simulink model "MotorCtrl_FOC_Physic"  (R2023b)
settings: Solver=FixedStepDiscrete  StartTime=0.0  StopTime=10  FixedStep=MC_Sim_BaseStep  RelTol=1e-3  EnableMultiTasking=on
values from neighbouring files (symbols this model uses):
  MC_MOS_DeadTime = 1.0E-6    [MotorControlDataDictionary_Math.sldd]    (also in MotorControlDataDictionary_Physic.sldd)
  MC_Motor_Mechinal_Inertia = 0.0103    [MotorControlDataDictionary_Math.sldd]    (also in MotorControlDataDictionary_Physic.sldd)
  MC_Motor_Phi = 0.0059190254913385806    [MotorControlDataDictionary_Math.sldd]    (also in MotorControlDataDictionary_Physic.sldd)
  MC_Motor_Rotor_Pn = 4.0    [MotorControlDataDictionary_Math.sldd]    (also in MotorControlDataDictionary_Physic.sldd)
  MC_Motor_Stator_Ld = 5.6345E-5    [MotorControlDataDictionary_Math.sldd]    (also in MotorControlDataDictionary_Physic.sldd)
  MC_Motor_Stator_Lq = 5.6345E-5    [MotorControlDataDictionary_Math.sldd]    (also in MotorControlDataDictionary_Physic.sldd)
  MC_Motor_Stator_Rs = 0.0286    [MotorControlDataDictionary_Math.sldd]    (also in MotorControlDataDictionary_Physic.sldd)
  MC_Param_CurrentPI_Ki = 0.0071879639914134473    [MotorControlDataDictionary_Math.sldd]    (also in MotorControlDataDictionary_Physic.sldd)
  MC_Param_CurrentPI_Kp = 0.283220860906427    [MotorControlDataDictionary_Math.sldd]    (also in MotorControlDataDictionary_Physic.sldd)
  MC_Param_CurrentPI_UdInteMax = 7.794228634059948    [MotorControlDataDictionary_Math.sldd]    (also in MotorControlDataDictionary_Physic.sldd)
  MC_Param_CurrentPI_UdInteMin = -7.794228634059948    [MotorControlDataDictionary_Math.sldd]    (also in MotorControlDataDictionary_Physic.sldd)
  MC_Param_CurrentPI_UdMax = 7.794228634059948    [MotorControlDataDictionary_Math.sldd]    (also in MotorControlDataDictionary_Physic.sldd)
  MC_Param_CurrentPI_UdMin = -7.794228634059948    [MotorControlDataDictionary_Math.sldd]    (also in MotorControlDataDictionary_Physic.sldd)
  MC_Param_CurrentPI_UqInteMax = 7.794228634059948    [MotorControlDataDictionary_Math.sldd]    (also in MotorControlDataDictionary_Physic.sldd)
  MC_Param_CurrentPI_UqInteMin = -7.794228634059948    [MotorControlDataDictionary_Math.sldd]    (also in MotorControlDataDictionary_Physic.sldd)
  MC_Param_CurrentPI_UqMax = 7.794228634059948    [MotorControlDataDictionary_Math.sldd]    (also in MotorControlDataDictionary_Physic.sldd)
  MC_Param_CurrentPI_UqMin = -7.794228634059948    [MotorControlDataDictionary_Math.sldd]    (also in MotorControlDataDictionary_Physic.sldd)
  MC_Param_Flux_Gamma = 750000.0    [MotorControlDataDictionary_Math.sldd]    (also in MotorControlDataDictionary_Physic.sldd)
  MC_Param_PhasetoReal = 500.0    [MotorControlDataDictionary_Math.sldd]    (also in MotorControlDataDictionary_Physic.sldd)
  MC_Param_SMO_CoffA = 0.97462064069571386    [MotorControlDataDictionary_Math.sldd]    (also in MotorControlDataDictionary_Physic.sldd)
  MC_Param_SMO_CoffB = 0.88739018546454884    [MotorControlDataDictionary_Math.sldd]    (also in MotorControlDataDictionary_Physic.sldd)
  MC_Param_SpeedCtrl_IdMax = 60.0    [MotorControlDataDictionary_Math.sldd]    (also in MotorControlDataDictionary_Physic.sldd)
  MC_Param_SpeedCtrl_IdMin = -60.0    [MotorControlDataDictionary_Math.sldd]    (also in MotorControlDataDictionary_Physic.sldd)
  MC_Param_SpeedCtrl_IqMax = 60.0    [MotorControlDataDictionary_Math.sldd]    (also in MotorControlDataDictionary_Physic.sldd)
  MC_Param_SpeedCtrl_IqMin = -60.0    [MotorControlDataDictionary_Math.sldd]    (also in MotorControlDataDictionary_Physic.sldd)
  MC_Param_SpeedPI_Ki = 0.57248683633241571    [MotorControlDataDictionary_Math.sldd]    (also in MotorControlDataDictionary_Physic.sldd)
  MC_Param_SpeedPI_Kp = 9.1114109857344836    [MotorControlDataDictionary_Math.sldd]    (also in MotorControlDataDictionary_Physic.sldd)
  MC_Param_SpeedtoTheta = 5.0E-5    [MotorControlDataDictionary_Math.sldd]    (also in MotorControlDataDictionary_Physic.sldd)
  MC_Param_SVPWM_DutyMax = 0.98    [MotorControlDataDictionary_Math.sldd]    (also in MotorControlDataDictionary_Physic.sldd)
  MC_Param_SVPWM_DutyMin = 0.02    [MotorControlDataDictionary_Math.sldd]    (also in MotorControlDataDictionary_Physic.sldd)
  MC_Param_SVPWM_SampleOffset1 = 0.02    [MotorControlDataDictionary_Math.sldd]    (also in MotorControlDataDictionary_Physic.sldd)
  MC_Param_SVPWM_SampleOffset2 = 0.015    [MotorControlDataDictionary_Math.sldd]    (also in MotorControlDataDictionary_Physic.sldd)
  MC_Param_SVPWM_SampleValid = 0.011999999999999999    [MotorControlDataDictionary_Math.sldd]    (also in MotorControlDataDictionary_Physic.sldd)
  MC_Sample_CurrentNoise = 1.0E-15    [MotorControlDataDictionary_Math.sldd]    (also in MotorControlDataDictionary_Physic.sldd)
  MC_Sample_VbusNoise = 1.0E-15    [MotorControlDataDictionary_Math.sldd]    (also in MotorControlDataDictionary_Physic.sldd)
  MC_Sim_BaseStep = 5.0E-8    [MotorControlDataDictionary_Math.sldd]    (also in MotorControlDataDictionary_Physic.sldd)
  MC_Sim_HFTStep = 5.0E-5    [MotorControlDataDictionary_Math.sldd]    (also in MotorControlDataDictionary_Physic.sldd)
  MC_Sim_MFTStep = 0.002    [MotorControlDataDictionary_Math.sldd]    (also in MotorControlDataDictionary_Physic.sldd)
libraries: simulink x17, nesl_utility x15, ee_lib x10, fl_lib x8
(part 2 of 3)

== system MotorCtrl_FOC_Physic/Hardware_Math/MotorHardware ==
  Load : Inport
  PWM : Inport  Port=2
  Current and Voltage Sensor (Three-Phase) : ee_lib/Sensors & Transducers/Current and Voltage Sensor (Three-Phase)  vMeasurementType=ee.enum.vmeasurement.ll  outputUnit=ee.enum.unit.si  SRated=100e6 A*V  VRated=24e3 V  I_specify=off  I_priority=None  I=[0, 0, 0] A  I_nominal_specify=off  I_nominal_unit=A  I_nominal_value=1  V_specify=off  V_priority=None  V=[0, 0, 0] V  V_nominal_specify=off  V_nominal_unit=V  V_nominal_value=1
      settings: InternalSimscapePortConfiguration="{\"Bottom\":[],\"Left\":[{\"id\":\"a1\",\"label\":\"a1\",\"type\":\"foundation.electrical.electrical\"},{\"id\":\"b1\",\"label\":\"b1\",\"type\":\"foundation.electrical.electrical\"},{\"id\":\"c1\",\"label\":\"c1\",\"type\":\"foundation.electrical.electrical\"}],\"Right\":[{\"id\":\"V_output\",\"label\":\"V\",\"type\":\"output\"},{\"id\":\"I_output\",\"label\":\"I\",\"type\":\"output\"},{\"id\":\"a2\",\"label\":\"a2\",\"type\":\"foundation.electrical.electrical\"},{\"id\":\"b2\",\"label\":\"b2\",\"type\":\"foundation.electrical.electrical\"},{\"id\":\"c2\",\"label\":\"c2\",\"type\":\"foundation.electrical.electrical\"}],\"Top\":[]}"
  Demux : Demux  Outputs=6
  Electrical Reference : fl_lib/Electrical/Electrical Elements/Electrical Reference
  MOSFET (Ideal, Switching){,1..5} (6 alike) : ee_lib/Semiconductors & Converters/MOSFET (Ideal, Switching)  port_option=ee.enum.controlport.ps  Rds=MC_MOS_Rds Ohm  Goff=MC_MOS_Cs 1/Ohm  Vth=MC_MOS_Threshold V  diode_param=ee.enum.converters.protectiondiode.none  diode_Vf=0.8 V  diode_Ron=0.001 Ohm  diode_Goff=1e-5 1/Ohm  diode_C=50e-9 F  diode_iRM=-235 A  diode_iF=300 A  diode_idot=-50 A/us  diode_trr_param=ee.enum.converters.diodeReverseParam.trr_factor  diode_trr_factor=3  diode_trr=15 us  diode_Qrr=1500 s*uA  ids_specify=off  ids_priority=None  ids=0 A  ids_nominal_specify=off  ids_nominal_unit=A  ids_nominal_value=1  vds_specify=off  vds_priority=None  vds=0 V  vds_nominal_specify=off  vds_nominal_unit=V  vds_nominal_value=1  vgs_specify=off  vgs_priority=None  vgs=0 V  vgs_nominal_specify=off  vgs_nominal_unit=V  vgs_nominal_value=1  thermal_loss_option=ee.enum.converters.thermalLossOption.constantvalues  Von_data=[0, 1.8, 3.2, 6, 10, 16; 0, 2, 5.5, 9.5, 15, 25] V  Tj=[298.15, 448.15] K  Iout_data=[0, 20, 40, 60, 80, 100] A  Eon_data=[0, 55.04, 124.57, 235.53, 362.12; 0, 71.25, 161.25, 304.88, 468.75] * 1e-6 J  Eoff_data=[0, 18, 30, 56.1, 76.5; 0, 22.5, 37.5, 70.13, 95.63] * 1e-6 J  Eon_data_3D=[zeros(2, 5, 3)] J  Eoff_data_3D=[zeros(2, 5, 3)] J  Tj_loss=[298.15, 448.15] K  Iout_data_loss=[0, 10, 20, 30, 40] A  tabulateWithVds=false  Vds_loss=[0, 150, 300] V  Eon_scalar=22.86e-3 J  Eoff_scalar=17.14e-3 J  Voff=300 V  Iout_scalar=600 A  useCurrentFromPreviousCycle=false  useVoltageFromPreviousCycle=false  diodeModelType=ee.enum.converters.diodeModelType.pwl  diodeTableType=ee.enum.diode.tableType.IfMat  diode_IfMat=[.07, .12, .19, 1.75, 4.24, 7.32, 11.2; .16, .3, .72, 2.14, 4.02, 6.35, 9.12] A  diode_VfMat=[.9, 1.15, 1.25, 1.5, 1.75, 2.17, 2.6, 2.85; .58, .68, .75, 1.1, 1.38, 1.77, 2.27, 2.7] V  diode_TjVec=[25, 125] degC  diode_VfVec=[.5, .7, .9, 1.3, 1.7, 2.1, 2.5] V  diode_IfVec=[.1, .2, .5, 1, 2, 4, 7, 10] A  diode_Vr=-600 V  diode_Ls=150 nH  diode_Erec=0.03 J  diode_rec_loss_model=ee.enum.diode.reverseRecoveryModel.fixed  diode_ErecVal=0 J  diode_scaleWithIandV=true  diode_ErecMat=zeros(2, 3) J  diode_TjrecVec=[298.15, 398.15] K  diode_IfrecVec=[.1, 1, 10] A  diode_IrecVal=10 A  diode_VrecVal=10 V  diode_tFilter=1 / 1000 / 100 s  thermal_network_parameterization=ee.enum.thermalNetworkTopology.external  Rth=[.03, .2] K/W  Rth_Cauer=[.03, .1, .2] K/W  Rth_Foster=[.03, .2] K/W  thermal_mass_parameterization=ee.enum.thermalNetwork.timeconstant  thermal_mass=[3, 25] J/K  thermal_mass_Cauer=[3, 10, 25] J/K  thermal_mass_Foster=[33, 50] J/K  thermal_time_constant=[.1, 5] s  thermal_time_constant_Cauer=[.1, 1, 5] s  thermal_time_constant_Foster=[1, 10] s  thermal_mass_initial_temperatures=[25, 25] degC  thermal_mass_initial_temperatures_Cauer=[25, 25, 25] degC  junction_thermal_mass=0.1 J/K  Tvec_initial_Foster=[25, 25, 25, 25] degC  no_thermal_network=0  junction_temperature_specify=off  junction_temperature_priority=None  junction_temperature=25 degC  junction_temperature_nominal_specify=off  junction_temperature_nominal_unit=degC  junction_temperature_nominal_value=1  Qj_specify=off  Qj_priority=None  Qj=0 W  Qj_nominal_specify=off  Qj_nominal_unit=W  Qj_nominal_value=1  accumulatedSwitchingLosses_specify=off  accumulatedSwitchingLosses_priority=None  accumulatedSwitchingLosses=0 J
  Mux : Mux  Inputs=3
  PMSM : ee_lib/Electromechanical/Permanent Magnet/PMSM  port_option=ee.enum.threePhasePort.expanded  winding_type=ee.enum.statorconnection.delta  machine_param=ee.enum.pmsm.parameterization.constant  nPolePairs=MC_Motor_Rotor_Pn  pmflux_param=ee.enum.pmflux.fluxlinkage  pm_flux_linkage=MC_Motor_Phi Wb  torque_constant=0.18 N*m/A  back_emf_constant=0.18 V*s/rad  stator_param=ee.enum.statorparam.LdLqL0  Ld=MC_Motor_Stator_Ld H  Lq=MC_Motor_Stator_Lq H  idVec=[-200, 0, 200] A  iqVec=[-200, 0, 200] A  LdMatrix=0.0002 * ones(3, 3) H  LqMatrix=0.0002 * ones(3, 3) H  PmMatrix=0.1 * ones(3, 3) Wb  ktMatrix=0.18 * ones(3, 3) N*m/A  keMatrix=0.18 * ones(3, 3) V*s/rad  L0=MC_Motor_Stator_L0 H  Ls=0.0002 H  Lm=-0.00002 H  Ms=0.00002 H  Rs=MC_Motor_Stator_Rs Ohm  zero_sequence=ee.enum.park.zerosequence.include  axes_param=ee.enum.rotorangle.daxis  loss_param=ee.enum.ironloss.none  losses_oc=[0, 0, 0] W  losses_sc=[0, 0, 0] W  f_losses=60 Hz  Isc_losses=95 A  J=MC_Motor_Mechinal_Inertia kg*m^2  lam=MC_Motor_Mechinal_Damp N*m*s/rad  i_d_specify=off  i_d_priority=None  i_d=0 A  i_d_nominal_specify=off  i_d_nominal_unit=A  i_d_nominal_value=1  i_q_specify=off  i_q_priority=None  i_q=0 A  i_q_nominal_specify=off  i_q_nominal_unit=A  i_q_nominal_value=1  torque_specify=off  torque_priority=None  torque=0 N*m  torque_nominal_specify=off  torque_nominal_unit=N*m  torque_nominal_value=1  angular_velocity_specify=off  angular_velocity_priority=High  angular_velocity=0 rpm  angular_velocity_nominal_specify=off  angular_velocity_nominal_unit=rpm  angular_velocity_nominal_value=1  angular_position_specify=on  angular_position_priority=High  angular_position=0 deg  angular_position_nominal_specify=off  angular_position_nominal_unit=deg  angular_position_nominal_value=1  alpha=3.93e-3 1/K  alpha_flux=-0.001 1/K  Tmeas=298.15 K  stator_thermal_mass=100 J/K  rotor_thermal_mass=200 J/K  Rm_percent_rotor=90  Rd_percent_rotor=30  temperatureA_specify=off  temperatureA_priority=High  temperatureA=25 degC  temperatureA_nominal_specify=off  temperatureA_nominal_unit=degC  temperatureA_nominal_value=1  temperatureB_specify=off  temperatureB_priority=High  temperatureB=25 degC  temperatureB_nominal_specify=off  temperatureB_nominal_unit=degC  temperatureB_nominal_value=1  temperatureC_specify=off  temperatureC_priority=High  temperatureC=25 degC  temperatureC_nominal_specify=off  temperatureC_nominal_unit=degC  temperatureC_nominal_value=1  temperatureR_specify=off  temperatureR_priority=High  temperatureR=25 degC  temperatureR_nominal_specify=off  temperatureR_nominal_unit=degC  temperatureR_nominal_value=1
      settings: InternalSimscapePortConfiguration="{\"Bottom\":[],\"Left\":[{\"id\":\"a\",\"label\":\"a\",\"type\":\"foundation.electrical.electrical\"},{\"id\":\"b\",\"label\":\"b\",\"type\":\"foundation.electrical.electrical\"},{\"id\":\"c\",\"label\":\"c\",\"type\":\"foundation.electrical.electrical\"}],\"Right\":[{\"id\":\"R\",\"label\":\"R\",\"type\":\"foundation.mechanical.rotational.rotational\"},{\"id\":\"C\",\"label\":\"C\",\"type\":\"foundation.mechanical.rotational.rotational\"}],\"Top\":[]}"
  PS-Simulink Converter{,1..3} (4 alike) : nesl_utility/PS-Simulink Converter  PhysicalDomain=network_engine_domain  SubClassName=ps_output  LeftPortType=input  RightPortType=output  PseudoPeriodic=off  Frequencies=[]  VectorFormat=inherit  Unit=inherit  AffineConversion=off
  Resistor : ee_lib/Passive/Resistor  R=0.001 Ohm  enable_R_tol=ee.enum.toleranceApplication.none  R_tol=5  tol_distribution=ee.enum.toleranceDistribution.uniform  nSigma=4  enable_operating_limits=ee.enum.enable.no  operating_limit_action=ee.enum.passive.reportOpLim.warn  power_rating=1 W  max_working_voltage=100 V  enable_faults=ee.enum.enable.no  fault_action=simscape.enum.assert.action.none  R_faulted=inf Ohm  fault_trigger=ee.enum.faults.faultTrigger.temporal  t_fault=1 s  max_permissible_current=1 A  t_fail_on_current=1 s  noise_mode=ee.enum.sources.noise.Disabled  Tdevice=25 degC  sample_time=1e-3 s  repeatability=ee.enum.ic.repeatability.notRepeatable  user_seed=0  auto_seed=3890346746  faulted_specify=off  faulted_priority=None  faulted=0  power_derating_T1=70 degC  power_derating_T2=155 degC  operating_temperature_range_vec=[-50, 150] degC  alpha=3.93e-3 1/K  Tmeas=25 degC  thermal_mass=100 J/K  temperature_specify=off  temperature_priority=High  temperature=298.15 K  temperature_nominal_specify=off  temperature_nominal_unit=K  temperature_nominal_value=1
  Simulink-PS Converter{,1..5} (6 alike) : nesl_utility/Simulink-PS Converter  PhysicalDomain=network_engine_domain  SubClassName=ps_input  LeftPortType=input  RightPortType=output  PseudoPeriodic=off  Frequencies=[]  NoiseDistribution=none  NoiseParameters=[]  Unit=1  AffineConversion=off  FilteringAndDerivatives=provide  SimscapeFilterOrder=1  InputFilterTimeConstant=0.001  UdotUserProvided=0
  Subsystem : Subsystem
  Voltage Sensor : fl_lib/Electrical/Electrical Sensors/Voltage Sensor
  Voltage Sensor1 : fl_lib/Electrical/Electrical Sensors/Voltage Sensor
  Voltage Source : ee_lib/Sources/Voltage Source  dc_voltage=MC_Input_Vdc V  ac_voltage=0 V  ac_shift=0 rad  ac_frequency=60 Hz  noise_mode=ee.enum.sources.noise.Disabled  PSD=0 V^2/Hz  sample_time=1e-3 s  repeatability=ee.enum.sources.repeatability.NotRepeatable  user_seed=0  auto_seed=3499211588  i_specify=off  i_priority=None  i=0 A  i_nominal_specify=off  i_nominal_unit=A  i_nominal_value=1  v_specify=off  v_priority=None  v=0 V  v_nominal_specify=off  v_nominal_unit=V  v_nominal_value=1
  Vabc : Outport
  Iabc : Outport  Port=2
  m : Outport  Port=3
  Vbus : Outport  Port=4
  Current : Outport  Port=5
  wires:
  Demux/1 -> Simulink-PS Converter/1
  PWM/1 -> Demux/1
  Demux/6 -> Simulink-PS Converter5/1
  Demux/5 -> Simulink-PS Converter4/1
  Demux/4 -> Simulink-PS Converter3/1
  Demux/3 -> Simulink-PS Converter2/1
  Demux/2 -> Simulink-PS Converter1/1
  Load/1 -> Subsystem/1(input0)
  PS-Simulink Converter/1 -> Current/1
  PS-Simulink Converter1/1 -> Vbus/1
  PS-Simulink Converter2/1 -> Vabc/1  "Vabc"
  PS-Simulink Converter3/1 -> Iabc/1  "Iabc"
  Subsystem/2(ThetaM) -> Mux/1
  Subsystem/1(Wm) -> Mux/2
  Subsystem/3(Te) -> Mux/3
  Mux/1 -> m/1
  connections:
  PMSM/LConn1 -- Current and Voltage Sensor (Three-Phase)/RConn3
  PMSM/LConn2 -- Current and Voltage Sensor (Three-Phase)/RConn4
  PMSM/LConn3 -- Current and Voltage Sensor (Three-Phase)/RConn5
  Subsystem/LConn1 -- PMSM/RConn1
  PMSM/RConn2 -- Subsystem/LConn2
  "MOSFET (Ideal, Switching)"/RConn2 -- "MOSFET (Ideal, Switching)1"/RConn1 -- Current and Voltage Sensor (Three-Phase)/LConn1
  Current and Voltage Sensor (Three-Phase)/LConn2 -- "MOSFET (Ideal, Switching)5"/RConn1 -- "MOSFET (Ideal, Switching)2"/RConn2
  Current and Voltage Sensor (Three-Phase)/LConn3 -- "MOSFET (Ideal, Switching)4"/RConn1 -- "MOSFET (Ideal, Switching)3"/RConn2
  Simulink-PS Converter/RConn1 -- "MOSFET (Ideal, Switching)"/LConn1
  "MOSFET (Ideal, Switching)1"/LConn1 -- Simulink-PS Converter1/RConn1
  "MOSFET (Ideal, Switching)2"/LConn1 -- Simulink-PS Converter2/RConn1
  "MOSFET (Ideal, Switching)5"/LConn1 -- Simulink-PS Converter3/RConn1
  "MOSFET (Ideal, Switching)3"/LConn1 -- Simulink-PS Converter4/RConn1
  "MOSFET (Ideal, Switching)4"/LConn1 -- Simulink-PS Converter5/RConn1
  Voltage Source/LConn1 -- Voltage Sensor/LConn1 -- "MOSFET (Ideal, Switching)3"/RConn1 -- "MOSFET (Ideal, Switching)2"/RConn1 -- "MOSFET (Ideal, Switching)"/RConn1
  Voltage Source/RConn1 -- Voltage Sensor1/RConn2 -- Resistor/RConn1 -- Voltage Sensor/RConn2 -- Electrical Reference/LConn1
  "MOSFET (Ideal, Switching)4"/RConn2 -- Voltage Sensor1/LConn1 -- Resistor/LConn1 -- "MOSFET (Ideal, Switching)5"/RConn2 -- "MOSFET (Ideal, Switching)1"/RConn2
  Voltage Sensor1/RConn1 -- PS-Simulink Converter/LConn1
  PS-Simulink Converter1/LConn1 -- Voltage Sensor/RConn1
  PS-Simulink Converter2/LConn1 -- Current and Voltage Sensor (Three-Phase)/RConn1
  PS-Simulink Converter3/LConn1 -- Current and Voltage Sensor (Three-Phase)/RConn2

== system MotorCtrl_FOC_Physic/Hardware_Math/PWMGenerate ==
  DutyABC : Inport
  SamplePoint : Inport  Port=2
  Compare To Constant : simulink/Logic and Bit Operations/Compare To Constant  relop=<=  const=1  OutDataTypeStr=boolean
  Data Type Conversion{,1,3..6} (6 alike) : DataTypeConversion  SaturateOnIntegerOverflow=off  RndMeth=Floor
  Data Type Conversion2 : DataTypeConversion  OutDataTypeStr=double  SaturateOnIntegerOverflow=off  RndMeth=Floor
  DeadTimeGenerate : Subsystem
  Mux : Mux  Inputs=6
  Rate Transition : RateTransition  OutPortSampleTime=MC_Sim_BaseStep
  Rate Transition1 : RateTransition  OutPortSampleTime=MC_Sim_BaseStep
  Relational Operator{,2..3,5} (4 alike) : RelationalOperator  OutDataTypeStr=boolean  RndMeth=Simplest  InputSameDT=off
  Relational Operator1 : RelationalOperator  Operator=<=  OutDataTypeStr=boolean  RndMeth=Simplest  InputSameDT=off
  Relational Operator4 : RelationalOperator  Operator=<=  OutDataTypeStr=boolean  RndMeth=Simplest  InputSameDT=off
  Relational Operator6 : RelationalOperator  Operator=<=  OutDataTypeStr=boolean  RndMeth=Simplest  InputSameDT=off
  Repeating Sequence : simulink/Sources/Repeating Sequence  rep_seq_t=[0 MC_Sim_HFTStep/2 MC_Sim_HFTStep]  rep_seq_y=[0 1 2]
  Repeating Sequence1 : simulink/Sources/Repeating Sequence  rep_seq_t=[0 MC_Sim_HFTStep/2 MC_Sim_HFTStep]  rep_seq_y=[2 1 0]
  Switch : Switch  Criteria=u2 > Threshold  SaturateOnIntegerOverflow=off  InputSameDT=off
  Gate : Outport
  CurrentSamplTrigger : Outport  Port=2
  wires:
  Data Type Conversion6/1 -> Mux/6  "PWMCDOWN"
  Data Type Conversion5/1 -> Mux/5  "PWMCUP"
  Data Type Conversion4/1 -> Mux/4  "PWMBDOWN"
  Data Type Conversion3/1 -> Mux/3  "PWMBUP"
  Data Type Conversion1/1 -> Mux/2  "PWMADOWN"
  Data Type Conversion/1 -> Mux/1  "PWMAUP"
  DeadTimeGenerate/6(GateCL) -> Relational Operator6/2
  DeadTimeGenerate/5(GateCH) -> Relational Operator5/2
  DeadTimeGenerate/4(GateBL) -> Relational Operator4/2
  DeadTimeGenerate/3(GateBH) -> Relational Operator2/2
  Relational Operator6/1 -> Data Type Conversion6/1
  Relational Operator5/1 -> Data Type Conversion5/1
  Relational Operator4/1 -> Data Type Conversion4/1
  Relational Operator2/1 -> Data Type Conversion3/1
  Relational Operator1/1 -> Data Type Conversion1/1
  Relational Operator/1 -> Data Type Conversion/1
  Repeating Sequence/1 -> Switch/1, Compare To Constant/1
  Repeating Sequence1/1 -> Switch/3
  DutyABC/1 -> DeadTimeGenerate/2(DutyABC)
  DeadTimeGenerate/1(GateAH) -> Relational Operator/2
  Switch/1 -> Rate Transition/1
  DeadTimeGenerate/2(GateAL) -> Relational Operator1/2
  Relational Operator3/1 -> Data Type Conversion2/1
  SamplePoint/1 -> Relational Operator3/2
  Data Type Conversion2/1 -> CurrentSamplTrigger/1  "CurrentSamplTrigger"
  Compare To Constant/1 -> Rate Transition1/1
  Mux/1 -> Gate/1  "Gate"
  Rate Transition/1 -> Relational Operator/1, Relational Operator1/1, Relational Operator3/1, Relational Operator6/1, Relational Operator5/1, Relational Operator4/1, Relational Operator2/1
  Rate Transition1/1 -> DeadTimeGenerate/1(FLag), Switch/2

== system MotorCtrl_FOC_Physic/Hardware_Math/VbusSample ==
  Vbus : Inport
  ADCOffset : Constant  Value=0  SampleTime=-1
  ADCQuality : Gain
  Add : Sum
  Data Type Conversion3 : DataTypeConversion  OutDataTypeStr=single  SaturateOnIntegerOverflow=off  RndMeth=Floor
  VbusSample : Outport
  wires:
  Vbus/1 -> Add/2
  Add/1 -> ADCQuality/1
  ADCQuality/1 -> Data Type Conversion3/1
  ADCOffset/1 -> Add/1
  Data Type Conversion3/1 -> VbusSample/1  "PhaseI"

== system MotorCtrl_FOC_Physic/Hardware_Math/currentSample ==
  SampleTrigger : Inport
  Current : Inport  Port=2
  getCurrentSample_ORS_Double : Subsystem  VariantControl=MC_Sample_Model==1 && MC_Sample_ORSType == 2
  getCurrentSample_ORS_Single : Subsystem  VariantControl=MC_Sample_Model==1 && MC_Sample_ORSType == 1
  getCurrentSample_TRS(Three) : Subsystem  VariantControl=MC_Sample_Model==3
  getCurrentSample_TRS(Two) : Subsystem  VariantControl=MC_Sample_Model==2
  SampleCurrent : Outport

== system MotorCtrl_FOC_Physic/MFTask/getCurrentLimit ==
  IdRef : Inport
  IqRef : Inport  Port=2
  Saturation : Saturate  UpperLimit=MC_Param_SpeedCtrl_IqMax  LowerLimit=MC_Param_SpeedCtrl_IqMin
  Saturation1 : Saturate  UpperLimit=MC_Param_SpeedCtrl_IdMax  LowerLimit=MC_Param_SpeedCtrl_IdMin
  Signal Copy : SignalConversion  OverrideOpt=off
  Signal Copy1 : SignalConversion  OverrideOpt=off
  IdRefLimit : Outport
  IqRefLimit : Outport  Port=2
  wires:
  IqRef/1 -> Saturation/1
  IdRef/1 -> Saturation1/1
  Signal Copy/1 -> IdRefLimit/1  "IdRefLimit"
  Signal Copy1/1 -> IqRefLimit/1  "IqRefLimit"
  Saturation/1 -> Signal Copy1/1
  Saturation1/1 -> Signal Copy/1

== system MotorCtrl_FOC_Physic/MFTask/piofSpeed ==
  SpeedTarget : Inport
  SpeedReal : Inport  Port=2
  Abs : Abs  SaturateOnIntegerOverflow=off
  Add : Sum
  Add1 : Sum
  Compare To Constant : simulink/Logic and Bit Operations/Compare To Constant  relop=>  const=0.01  OutDataTypeStr=boolean
  Constant : Constant  Value=0  OutDataTypeStr=single
  Constant1 : Constant  Value=0  OutDataTypeStr=single
  Delay One Step : Delay  DelayLength=1
  Gain : Gain  Gain=MC_Param_SpeedPI_Kp
  Gain1 : Gain  Gain=MC_Param_SpeedPI_Ki
  Saturation : Saturate  UpperLimit=50  LowerLimit=-50
  Saturation1 : Saturate  UpperLimit=50  LowerLimit=-50
  Subtract : Sum  Inputs=+-
  Switch : Switch  Criteria=u2 > Threshold  SaturateOnIntegerOverflow=off  InputSameDT=off
  IdRef : Outport
  IqRef : Outport  Port=2
  wires:
  Add/1 -> Saturation/1, Delay One Step/1
  Subtract/1 -> Switch/1, Abs/1, Gain/1
  Gain1/1 -> Add/1
  Saturation/1 -> Add1/2
  Delay One Step/1 -> Add/2
  Gain/1 -> Add1/1
  Compare To Constant/1 -> Switch/2
  Add1/1 -> Saturation1/1
  Abs/1 -> Compare To Constant/1
  Constant/1 -> Switch/3
  SpeedReal/1 -> Subtract/2
  Saturation1/1 -> IqRef/1  "IqRef"
  SpeedTarget/1 -> Subtract/1
  Switch/1 -> Gain1/1
  Constant1/1 -> IdRef/1  "IdRef"

== system MotorCtrl_FOC_Physic/MFTask/smcofSpeed ==
  SpeedTarget : Inport
  SpeedReal : Inport  Port=2
  Add : Sum
  Add1 : Sum
  Add2 : Sum
  Constant : Constant  Value=0  OutDataTypeStr=single
  Delay One Step : Delay  DelayLength=1
  Delay One Step1 : Delay  DelayLength=1
  Gain : Gain  Gain=1/MC_Sim_MFTStep
  Gain1 : Gain  Gain=200
  Gain2 : Gain  Gain=50
  Gain3 : Gain  Gain=MC_Sim_MFTStep*1*MC_Motor_Mechinal_Inertia/(3*MC_Motor_Phi*MC_Motor_Rotor_Pn)
  Saturation : Saturate  UpperLimit=2  LowerLimit=-2
  Subtract : Sum  Inputs=+-
  Subtract1 : Sum  Inputs=+-
  IdRef : Outport
  IqRef : Outport  Port=2
  wires:
  SpeedTarget/1 -> Subtract/1
  SpeedReal/1 -> Subtract/2
  Subtract/1 -> Delay One Step/1, Subtract1/1, Add/1  "E1"
  Delay One Step/1 -> Subtract1/2
  Subtract1/1 -> Gain/1
  Gain/1 -> Add/2, Gain2/1  "E2"
  Add/1 -> Saturation/1  "S"
  Saturation/1 -> Gain1/1  "sign(S)"
  Gain1/1 -> Add1/1
  Gain2/1 -> Add1/2
  Add1/1 -> Gain3/1  "IqRef_dot"
  Gain3/1 -> Add2/1
  Add2/1 -> IqRef/1, Delay One Step1/1  "IqRef"
  Delay One Step1/1 -> Add2/2
  Constant/1 -> IdRef/1  "IdRef"

== system MotorCtrl_FOC_Physic/svpwm_OM/getVoltageExchange ==
  Valpha : Inport
  Vbeta : Inport  Port=2
  Vdc : Inport  Port=3
  Add : Sum
  Add1 : Sum
  Divide : Product  Inputs=*/
  Divide1 : Product  Inputs=*/
  Gain : Gain  Gain=-1/2
  Gain1 : Gain  Gain=sqrt(3)/2
  Gain2 : Gain  Gain=-1
  Relational Operator : RelationalOperator  OutDataTypeStr=boolean  RndMeth=Simplest  InputSameDT=off
  Relational Operator1 : RelationalOperator  OutDataTypeStr=boolean  RndMeth=Simplest  InputSameDT=off
  Relational Operator2 : RelationalOperator  Operator=<=  OutDataTypeStr=boolean  RndMeth=Simplest  InputSameDT=off
  Relational Operator3 : RelationalOperator  Operator=<=  OutDataTypeStr=boolean  RndMeth=Simplest  InputSameDT=off
  Signal Copy : SignalConversion  OverrideOpt=off
  Subtract : Sum  Inputs=+-
  Switch{,1..3} (4 alike) : Switch  Criteria=u2 > Threshold  SaturateOnIntegerOverflow=off  InputSameDT=off
  getSectorN : Subsystem  Commented=on
  Va : Outport
  Vb : Outport  Port=2
  Vc : Outport  Port=3
  Vmed : Outport  Port=4
  wires:
  Gain2/1 -> Vmed/1  "Vmed"
  Add1/1 -> Gain2/1
  Relational Operator2/1 -> Switch2/2
  Switch2/1 -> Relational Operator3/1, Switch3/1
  Relational Operator3/1 -> Switch3/2
  Switch3/1 -> Add1/2  "Vmin"
  Relational Operator/1 -> Switch/2
  Switch/1 -> Switch1/1, Relational Operator1/1
  Relational Operator1/1 -> Switch1/2
  Switch1/1 -> Add1/1  "Vmax"
  Signal Copy/1 -> Va/1, Relational Operator/1, Switch/1, Relational Operator2/1, Switch2/1  "Va"
  Divide/1 -> Signal Copy/1, Gain/1
  Divide1/1 -> Gain1/1
  Gain/1 -> Subtract/1, Add/1
  Gain1/1 -> Add/2, Subtract/2
  Add/1 -> Vb/1, Relational Operator/2, Switch/3, Relational Operator2/2, Switch2/3  "Vb"
  Subtract/1 -> Vc/1, Switch1/3, Relational Operator1/2, Switch3/3, Relational Operator3/2  "Vc"
  Vdc/1 -> Divide1/2, Divide/2
  Vbeta/1 -> Divide1/1
  Valpha/1 -> Divide/1

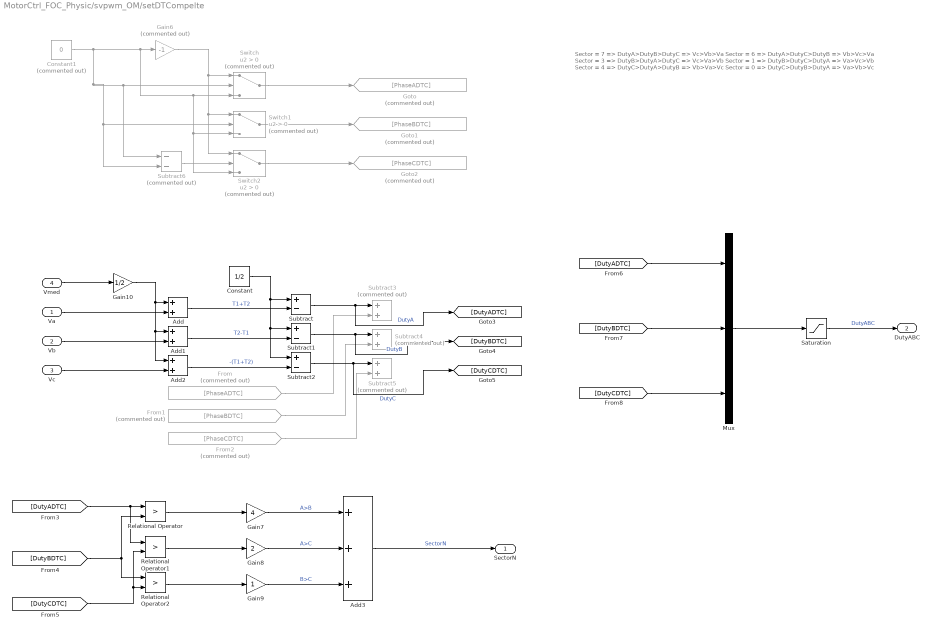
== system MotorCtrl_FOC_Physic/svpwm_OM/setDTCompelte ==
  note: Sector = 7 => DutyA>DutyB>DutyC => Vc>Vb>Va
      | Sector = 6 => DutyA>DutyC>DutyB => Vb>Vc>Va
      | Sector = 3 => DutyB>DutyA>DutyC => Vc>Va>Vb
      | Sector = 1 => DutyB>DutyC>DutyA => Va>Vc>Vb
      | Sector = 4 => DutyC>DutyA>DutyB => Vb>Va>Vc
      | Sector = 0 => DutyC>DutyB>DutyA => Va>Vb>Vc
  Va : Inport
  Vb : Inport  Port=2
  Vc : Inport  Port=3
  Vmed : Inport  Port=4
  Add : Sum
  Add1 : Sum
  Add2 : Sum
  Add3 : Sum  Inputs=+++
  Constant : Constant  Value=1/2  OutDataTypeStr=single
  Constant1 : Constant  Commented=on  Value=0  OutDataTypeStr=single
  From : From  Commented=on  GotoTag=PhaseADTC
  From1 : From  Commented=on  GotoTag=PhaseBDTC
  From2 : From  Commented=on  GotoTag=PhaseCDTC
  Gain10 : Gain  Gain=1/2
  Gain6 : Gain  Commented=on  Gain=-1
  Gain7 : Gain  Gain=4  OutDataTypeStr=single  RndMeth=Simplest
  Gain8 : Gain  Gain=2  OutDataTypeStr=single  RndMeth=Simplest
  Gain9 : Gain  OutDataTypeStr=single  RndMeth=Simplest
  Goto : Goto  Commented=on  GotoTag=PhaseADTC
  Goto1 : Goto  Commented=on  GotoTag=PhaseBDTC
  Goto2 : Goto  Commented=on  GotoTag=PhaseCDTC
  Mux : Mux  Inputs=3
  Relational Operator : RelationalOperator  Operator=>  OutDataTypeStr=boolean  RndMeth=Simplest  InputSameDT=off
  Relational Operator1 : RelationalOperator  Operator=>  OutDataTypeStr=boolean  RndMeth=Simplest  InputSameDT=off
  Relational Operator2 : RelationalOperator  Operator=>  OutDataTypeStr=boolean  RndMeth=Simplest  InputSameDT=off
  Saturation : Saturate  UpperLimit=MC_Param_SVPWM_DutyMax  LowerLimit=MC_Param_SVPWM_DutyMin
      settings: AttributesFormatString=|
      | OutputMax = %<UpperLimit>
      | OutputMin = %<LowerLimit>
  Subtract : Sum  Inputs=+-
  Subtract1 : Sum  Inputs=+-
  Subtract2 : Sum  Inputs=+-
  Subtract3 : Sum  Commented=on
  Subtract4 : Sum  Commented=on
  Subtract5 : Sum  Commented=on
  Subtract6 : Sum  Commented=on  Inputs=--
  Switch : Switch  Commented=on  Criteria=u2 > Threshold  SaturateOnIntegerOverflow=off  InputSameDT=off
  Switch1 : Switch  Commented=on  Criteria=u2 > Threshold  SaturateOnIntegerOverflow=off  InputSameDT=off
  Switch2 : Switch  Commented=on  Criteria=u2 > Threshold  SaturateOnIntegerOverflow=off  InputSameDT=off
  SectorN : Outport
  DutyABC : Outport  Port=2
  wires:
  Saturation/1 -> DutyABC/1  "DutyABC"
  Mux/1 -> Saturation/1
  Gain10/1 -> Add/1, Add1/1, Add2/1
  Add3/1 -> SectorN/1  "SectorN"
  Gain7/1 -> Add3/1  "A>B"
  Gain9/1 -> Add3/3  "B>C"
  Gain8/1 -> Add3/2  "A>C"
  Relational Operator2/1 -> Gain9/1
  Relational Operator1/1 -> Gain8/1
  Relational Operator/1 -> Gain7/1
  [DutyCDTC] -> Relational Operator1/2, Relational Operator2/2
  [DutyADTC] -> Relational Operator/1, Relational Operator1/1
  [DutyBDTC] -> Relational Operator2/1, Relational Operator/2
  From2/1 -> Subtract5/2
  From1/1 -> Subtract4/2
  From/1 -> Subtract3/2
  Switch2/1 -> Goto2/1
  Switch1/1 -> Goto1/1
  Switch/1 -> Goto/1
  Subtract6/1 -> Switch2/2
  Constant1/1 -> Switch1/2, Subtract6/2, Switch/2, Subtract6/1, Gain6/1, Switch/3, Switch1/3, Switch2/3
  Gain6/1 -> Switch/1, Switch1/1, Switch2/1
  Subtract2/1 -> [DutyCDTC], Subtract5/1  "DutyC"
  Subtract1/1 -> [DutyBDTC], Subtract4/1  "DutyB"
  Subtract/1 -> [DutyADTC], Subtract3/1  "DutyA"
  Constant/1 -> Subtract/1, Subtract1/1, Subtract2/1
  Add1/1 -> Subtract1/2  "T2-T1"
  Add2/1 -> Subtract2/2  "-(T1+T2)"
  Add/1 -> Subtract/2  "T1+T2"
  Vc/1 -> Add2/2
  Vb/1 -> Add1/2
  Vmed/1 -> Gain10/1
  Va/1 -> Add/2
  [DutyADTC] -> Mux/1
  [DutyBDTC] -> Mux/2
  [DutyCDTC] -> Mux/3

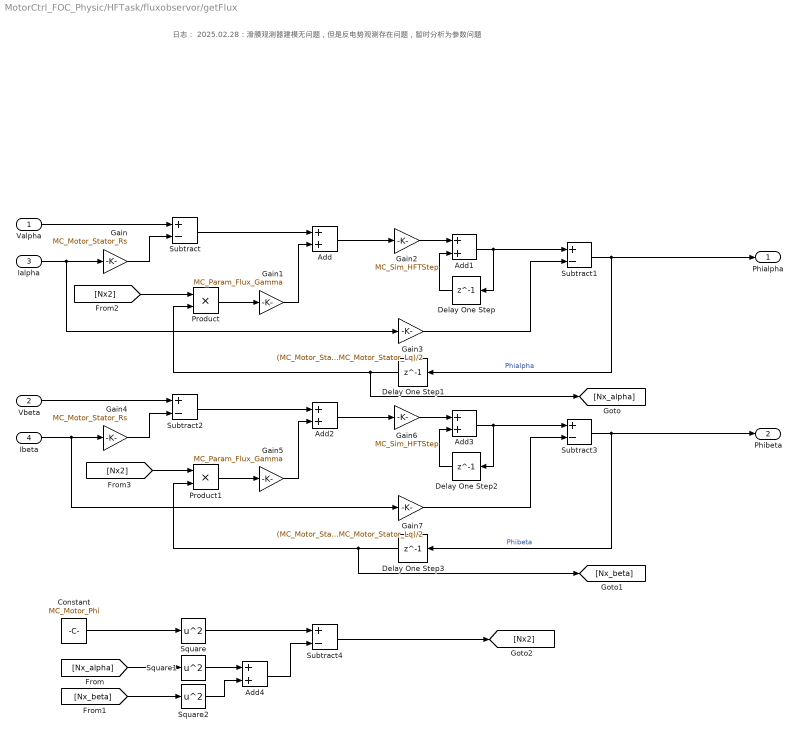
== system MotorCtrl_FOC_Physic/HFTask/fluxobservor/getFlux ==
  note: 日志：
      | 2025.02.28：滑膜观测器建模无问题，但是反电势观测存在问题，暂时分析为参数问题
  Valpha : Inport
  Vbeta : Inport  Port=2
  Ialpha : Inport  Port=3
  Ibeta : Inport  Port=4
  Add{,1..4} (5 alike) : Sum
  Constant : Constant  Value=MC_Motor_Phi  OutDataTypeStr=single
  Delay One Step{,1..3} (4 alike) : Delay  DelayLength=1
  Gain : Gain  Gain=MC_Motor_Stator_Rs
  Gain1 : Gain  Gain=MC_Param_Flux_Gamma  OutDataTypeStr=single  RndMeth=Simplest
  Gain2 : Gain  Gain=MC_Sim_HFTStep  OutDataTypeStr=single  RndMeth=Simplest
  Gain3 : Gain  Gain=(MC_Motor_Stator_Ld+MC_Motor_Stator_Lq)/2  OutDataTypeStr=single  RndMeth=Simplest
  Gain4 : Gain  Gain=MC_Motor_Stator_Rs
  Gain5 : Gain  Gain=MC_Param_Flux_Gamma  OutDataTypeStr=single  RndMeth=Simplest
  Gain6 : Gain  Gain=MC_Sim_HFTStep
  Gain7 : Gain  Gain=(MC_Motor_Stator_Ld+MC_Motor_Stator_Lq)/2  OutDataTypeStr=single  RndMeth=Simplest
  Product : Product
  Product1 : Product
  Square : Math  Operator=square
  Square1 : Math  Operator=square
  Square2 : Math  Operator=square
  Subtract{,1..4} (5 alike) : Sum  Inputs=+-
  Phialpha : Outport
  Phibeta : Outport  Port=2
  wires:
  Valpha/1 -> Subtract/1
  Ialpha/1 -> Gain3/1, Gain/1
  Gain/1 -> Subtract/2
  Subtract/1 -> Add/1
  Gain1/1 -> Add/2
  Add/1 -> Gain2/1
  Add1/1 -> Subtract1/1, Delay One Step/1
  Delay One Step/1 -> Add1/2
  Gain2/1 -> Add1/1
  Gain3/1 -> Subtract1/2
  Subtract1/1 -> Phialpha/1, Delay One Step1/1  "Phialpha"
  Product/1 -> Gain1/1
  Delay One Step1/1 -> [Nx_alpha], Product/2
  Delay One Step3/1 -> [Nx_beta], Product1/2
  Product1/1 -> Gain5/1
  Subtract3/1 -> Phibeta/1, Delay One Step3/1  "Phibeta"
  Gain7/1 -> Subtract3/2
  Gain6/1 -> Add3/1
  Delay One Step2/1 -> Add3/2
  Add3/1 -> Delay One Step2/1, Subtract3/1
  Add2/1 -> Gain6/1
  Gain5/1 -> Add2/2
  Subtract2/1 -> Add2/1
  Gain4/1 -> Subtract2/2
  Ibeta/1 -> Gain4/1, Gain7/1
  Vbeta/1 -> Subtract2/1
  Constant/1 -> Square/1
  [Nx_alpha] -> Square1/1
  [Nx_beta] -> Square2/1
  Square1/1 -> Add4/1
  Square2/1 -> Add4/2
  Square/1 -> Subtract4/1
  Add4/1 -> Subtract4/2
  Subtract4/1 -> [Nx2]
  [Nx2] -> Product/1
  [Nx2] -> Product1/1

== system MotorCtrl_FOC_Physic/HFTask/fluxobservor/getSpeedandTheta ==
  Phialpha : Inport
  Phibeta : Inport  Port=2
  Add : Sum
  Add1 : Sum
  Add2 : Sum
  Constant : Constant  Value=2*pi  OutDataTypeStr=single
  Delay One Step : Delay  DelayLength=1
  Delay One Step2 : Delay  DelayLength=1
  Gain : Gain  Gain=1/MC_Motor_Phi
  Gain1 : Gain  Gain=2*sqrt(2)/2*100
  Gain2 : Gain  Gain=100^2*MC_Sim_HFTStep
  Gain3 : Gain  Gain=MC_Param_SpeedtoTheta  OutDataTypeStr=single  RndMeth=Simplest
  Gain4 : Gain  Gain=1/MC_Motor_Phi
  Gain5 : Gain  Gain=30/(pi*MC_Motor_Rotor_Pn)  OutDataTypeStr=single  RndMeth=Simplest
  Mod : Math  Operator=mod
  Product : Product
  Product1 : Product
  Sin : Trigonometry  OutputSignalType=real
  Sin1 : Trigonometry  Operator=cos  OutputSignalType=real
  Subtract : Sum  Inputs=+-
  Speed : Outport
  Theta : Outport  Port=2
  wires:
  [Theta_Last] -> Sin/1, Sin1/1
  Add1/1 -> Gain5/1, Gain3/1  "SpeedFlux"
  Mod/1 -> Delay One Step2/1, Theta/1  "ThetaFlux"
  Delay One Step2/1 -> [Theta_Last], Add2/2
  Constant/1 -> Mod/2
  Add2/1 -> Mod/1
  Gain3/1 -> Add2/1
  Subtract/1 -> Gain1/1, Gain2/1  "FluxErr"
  Gain1/1 -> Add1/1
  Delay One Step/1 -> Add/2
  Add/1 -> Add1/2, Delay One Step/1
  Gain2/1 -> Add/1
  Product1/1 -> Subtract/2  "FluxSin"
  Product/1 -> Subtract/1  "FluxCos"
  Sin/1 -> Product1/2
  Sin1/1 -> Product/2
  Phibeta/1 -> Gain/1
  Phialpha/1 -> Gain4/1
  Gain/1 -> Product/1
  Gain4/1 -> Product1/1
  Gain5/1 -> Speed/1  "SpeedFlux_RPM"

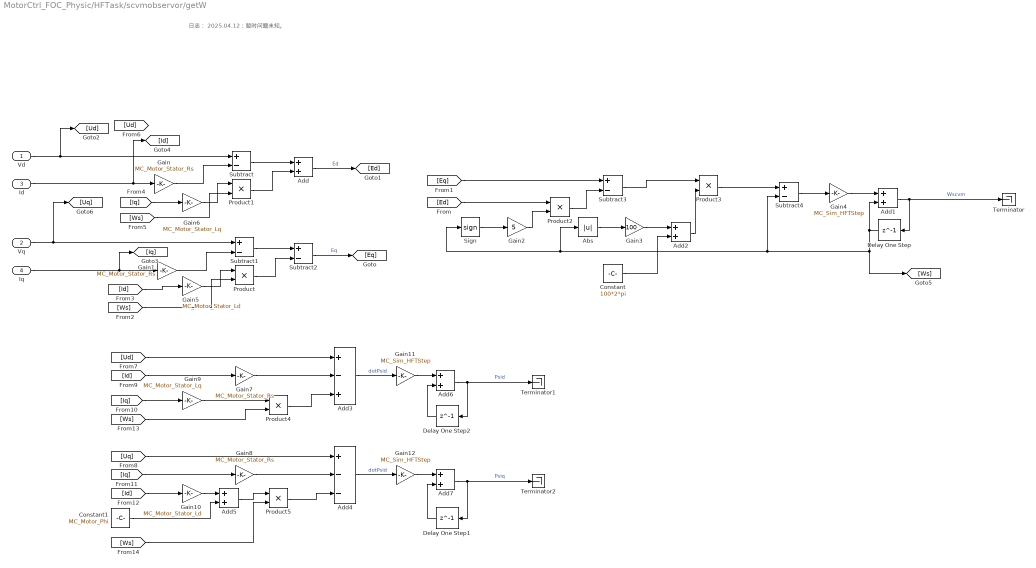
== system MotorCtrl_FOC_Physic/HFTask/scvmobservor/getW ==
  note: 日志：
      | 2025.04.12：暂时问题未知。
  Vd : Inport
  Vq : Inport  Port=2
  Id : Inport  Port=3
  Iq : Inport  Port=4
  Abs : Abs  SaturateOnIntegerOverflow=off
  Add{,1..2,5..7} (6 alike) : Sum
  Add3 : Sum  Inputs=+-+
  Add4 : Sum  Inputs=+--
  Constant : Constant  Value=100*2*pi  OutDataTypeStr=single
  Constant1 : Constant  Value=MC_Motor_Phi  OutDataTypeStr=single
  Delay One Step : Delay  DelayLength=1
  Delay One Step1 : Delay  DelayLength=1
  Delay One Step2 : Delay  DelayLength=1
  Gain{,1,7..8} (4 alike) : Gain  Gain=MC_Motor_Stator_Rs
  Gain10 : Gain  Gain=MC_Motor_Stator_Ld
  Gain11 : Gain  Gain=MC_Sim_HFTStep
  Gain12 : Gain  Gain=MC_Sim_HFTStep
  Gain2 : Gain  Gain=5
  Gain3 : Gain  Gain=100
  Gain4 : Gain  Gain=MC_Sim_HFTStep
  Gain5 : Gain  Gain=MC_Motor_Stator_Ld
  Gain6 : Gain  Gain=MC_Motor_Stator_Lq
  Gain9 : Gain  Gain=MC_Motor_Stator_Lq
  Product{,1..5} (6 alike) : Product
  Sign : Signum
  Subtract{,1..4} (5 alike) : Sum  Inputs=+-
  Terminator : Terminator
  Terminator1 : Terminator
  Terminator2 : Terminator
  wires:
  Id/1 -> [Id], Gain/1
  Gain/1 -> Subtract/2
  Subtract/1 -> Add/1
  Add/1 -> [Ed]  "Ed"
  Gain1/1 -> Subtract1/2
  Iq/1 -> [Iq], Gain1/1
  Vq/1 -> Subtract1/1, [Uq]
  Subtract1/1 -> Subtract2/1
  Product/1 -> Subtract2/2
  Product1/1 -> Add/2
  Subtract2/1 -> [Eq]  "Eq"
  [Ed] -> Product2/1
  Gain2/1 -> Product2/2
  Sign/1 -> Gain2/1
  [Eq] -> Subtract3/1
  Product2/1 -> Subtract3/2
  Subtract3/1 -> Product3/1
  Product3/1 -> Subtract4/1
  Gain4/1 -> Add1/1
  Add1/1 -> Delay One Step/1, Terminator/1  "Wscvm"
  Delay One Step/1 -> [Ws], Subtract4/2, Abs/1, Sign/1, Add1/2
  Subtract4/1 -> Gain4/1
  [Id] -> Gain5/1
  Gain5/1 -> Product/1
  [Ws] -> Product/2
  Gain6/1 -> Product1/1
  [Iq] -> Gain6/1
  [Ws] -> Product1/2
  Abs/1 -> Gain3/1
  Add2/1 -> Product3/2
  Gain3/1 -> Add2/1
  Constant/1 -> Add2/2
  Vd/1 -> Subtract/1, [Ud]
  [Id] -> Gain7/1
  [Iq] -> Gain8/1
  [Ud] -> Add3/1
  Gain7/1 -> Add3/2
  Gain8/1 -> Add4/2
  [Uq] -> Add4/1
  [Ws] -> Product4/2
  Product4/1 -> Add3/3
  Product5/1 -> Add4/3
  [Iq] -> Gain9/1
  Gain9/1 -> Product4/1
  [Id] -> Gain10/1
  Gain10/1 -> Add5/1
  Constant1/1 -> Add5/2
  Add5/1 -> Product5/1
  [Ws] -> Product5/2
  Add3/1 -> Gain11/1  "dotPsid"
  Add4/1 -> Gain12/1  "dotPsid"
  Add7/1 -> Terminator2/1, Delay One Step1/1  "Psiq"
  Delay One Step1/1 -> Add7/2
  Add6/1 -> Terminator1/1, Delay One Step2/1  "Psid"
  Delay One Step2/1 -> Add6/2
  Gain11/1 -> Add6/1
  Gain12/1 -> Add7/1

== system MotorCtrl_FOC_Physic/HFTask/smo/getE ==
  note: 日志：
      | 2025.02.28：滑膜观测器建模无问题，但是反电势观测存在问题，暂时分析为参数问题
  Valpha : Inport
  Vbeta : Inport  Port=2
  Ialpha : Inport  Port=3
  Ibeta : Inport  Port=4
  Add : Sum  Inputs=--+
  Add1 : Sum
  Add2 : Sum  Inputs=+--
  Add3 : Sum
  Delay One Step{,1..3} (4 alike) : Delay  DelayLength=1
  Gain{,4,6,8} (4 alike) : Gain  Gain=MC_Param_SMO_CoffB
  Gain3 : Gain  Gain=MC_Param_SMO_CoffA
  Gain7 : Gain  Gain=MC_Param_SMO_CoffA
  Saturation : Saturate  UpperLimit=100  LowerLimit=-100
  Saturation1 : Saturate  UpperLimit=100  LowerLimit=-100
  Subtract : Sum  Inputs=+-
  Subtract1 : Sum  Inputs=-+
  Ealpha : Outport
  Ebeta : Outport  Port=2
  wires:
  Valpha/1 -> Gain/1
  Add1/1 -> Subtract/1, Delay One Step/1  "Ialpha_Ob"
  Ialpha/1 -> Subtract/2
  Gain/1 -> Add/3
  Gain3/1 -> Add/2
  Gain4/1 -> Add/1
  Delay One Step1/1 -> [Ealpha_SMO]
  [Ialpha_SMO] -> Gain3/1
  [Ealpha_SMO] -> Gain4/1
  Subtract/1 -> Saturation/1  "Ialpha_ob-Ialpha"
  Saturation/1 -> Ealpha/1, Delay One Step1/1  "Ealpha"
  Gain6/1 -> Add2/1
  Gain7/1 -> Add2/2
  Gain8/1 -> Add2/3
  Vbeta/1 -> Gain6/1
  Add/1 -> Add1/1  "dotIalpha_ob"
  Delay One Step/1 -> Add1/2, [Ialpha_SMO]
  Add2/1 -> Add3/2  "dotIbeta_ob"
  Add3/1 -> Subtract1/2, Delay One Step2/1  "Ibeta_Ob"
  Delay One Step2/1 -> [Ibeta_SMO], Add3/1
  Ibeta/1 -> Subtract1/1
  Subtract1/1 -> Saturation1/1  "Ibeta_ob-Ibeta"
  Saturation1/1 -> Ebeta/1, Delay One Step3/1  "Ebeta"
  Delay One Step3/1 -> [Ebeta_SMO]
  [Ibeta_SMO] -> Gain7/1
  [Ebeta_SMO] -> Gain8/1

== system MotorCtrl_FOC_Physic/HFTask/smo/getSpeedandTheta ==
  note: 日志：
      | 2025.03.19：反电势正负号识别错误，改正后可以使用
  Ealpha : Inport
  Ebeta : Inport  Port=2
  Add : Sum
  Add1 : Sum
  Add2 : Sum
  Constant : Constant  Value=2*pi  OutDataTypeStr=single
  Delay One Step : Delay  DelayLength=1
  Delay One Step2 : Delay  DelayLength=1
  Gain : Gain  Gain=-1
  Gain1 : Gain  Gain=2*sqrt(2)/2*100
  Gain2 : Gain  Gain=100^2*MC_Sim_HFTStep
  Gain3 : Gain  Gain=MC_Param_SpeedtoTheta
  Gain5 : Gain  Gain=30/(pi*MC_Motor_Rotor_Pn)  OutDataTypeStr=single  RndMeth=Simplest
  Mod : Math  Operator=mod
  Product : Product
  Product1 : Product
  Sin : Trigonometry  OutputSignalType=real
  Sin1 : Trigonometry  Operator=cos  OutputSignalType=real
  Subtract : Sum  Inputs=+-
  Speed : Outport
  Theta : Outport  Port=2
  wires:
  Sin1/1 -> Product/2
  Sin/1 -> Product1/2
  Gain2/1 -> Add/1
  Add/1 -> Delay One Step/1, Add1/2
  Delay One Step/1 -> Add/2
  Gain1/1 -> Add1/1
  Subtract/1 -> Gain2/1, Gain1/1  "SMOErr"
  Gain3/1 -> Add2/1
  Add2/1 -> Mod/1
  Constant/1 -> Mod/2
  Delay One Step2/1 -> Add2/2, [Theta_Last]
  Mod/1 -> Theta/1, Delay One Step2/1  "ThetaSMO"
  Add1/1 -> Gain5/1, Gain3/1  "SpeedSmo"
  [Theta_Last] -> Sin1/1, Sin/1
  Gain/1 -> Product1/1
  Ebeta/1 -> Gain/1
  Ealpha/1 -> Product/1
  Product/1 -> Subtract/1  "SMOSin"
  Product1/1 -> Subtract/2  "SMOCos"
  Gain5/1 -> Speed/1  "SpeedSMO_RPM"
